simulink model "modulation"  (R2019b)
settings: Solver=ode23t  StartTime=0.0  StopTime=0.008  MaxStep=1e-6  RelTol=1e-3
libraries: powerlib x1
settings Model: Creator=Lenovo  LastModifiedBy=Lenovo

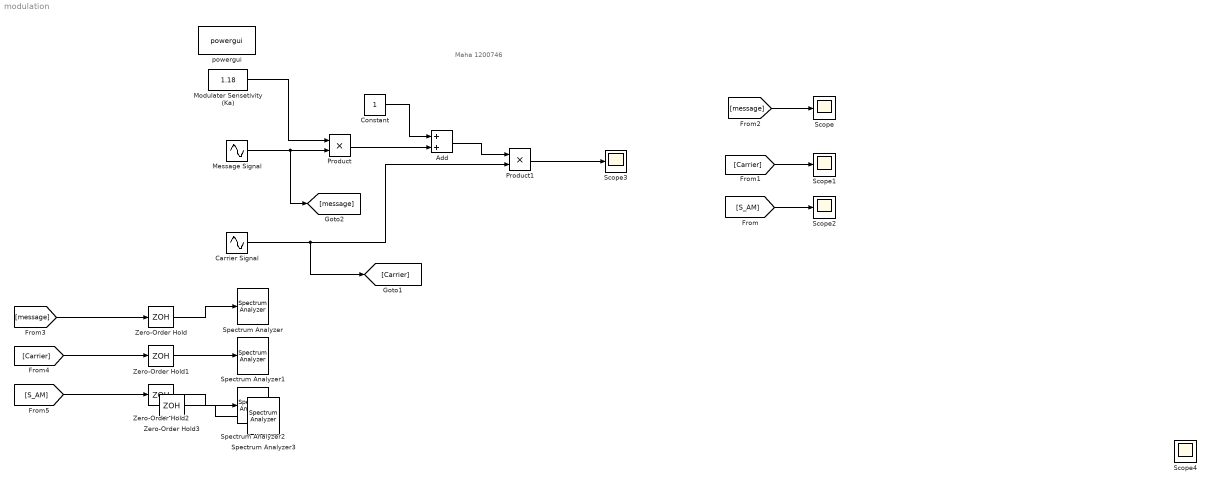
== system modulation ==
  note: Maha 1200746
  Add : Sum
  Carrier Signal : Sin  Frequency=2*pi*15000  SampleTime=0
  Constant : Constant
  Message Signal : Sin  Amplitude=0.85  Frequency=2*pi*1000  SampleTime=0
  Modulater Sensetivity (Ka) : Constant  Value=1.18
  Product : Product
  Product1 : Product
  Scope{,1..4} (5 alike) : Scope
  Spectrum Analyzer{,1..3} (4 alike) : SpectrumAnalyzer
  Zero-Order Hold : ZeroOrderHold  SampleTime=1/(10*1e3)
  Zero-Order Hold1 : ZeroOrderHold  SampleTime=1/(10*15e3)
  Zero-Order Hold2 : ZeroOrderHold  SampleTime=1/(10*15e3)
  Zero-Order Hold3 : ZeroOrderHold  SampleTime=1/(10*15e3)
  powergui : powerlib/powergui  Priority=1  SimulationMode=Continuous  SampleTime=50e-6  frequency=60  Iterations=50  frequencyindice=60  Pbase=100e6  ErrMax=1e-4  UnitsV=kV  UnitsW=MW  buscounter=0  FunctionMessages=off  echomessages=off  EnableUseOfTLC=off  CurrentSourceSwitches=off  DisableSnubberDevices=off  DisableRonSwitches=off  DisableVfSwitches=off  DisplayEquations=off  AutomaticDiscreteSolvers=off  SolverType=Tustin/Backward Euler (TBE)  Interpol=off  ExternalGateDelay=off  methode=off  Ts=100  x0status=blocks  SPID=on  SwTol=0  HookPort=off  NonlinearTolerance=1e-4  nMaxIteration=100  ContinueOnMaxIteration=off  RestoreLinks=warning  ResistiveCurrentMeasurement=off  Frange=[0:2:500]  Ylog=off  Xlog=on  ShowGrid=off  save=off  variable=ZData  structure=0  ZoomFFT=off  StartTime=0.0  cycles=1  DisplayStyle=1  fundamental=60  FreqAxis=off  MaxFrequency=1000  frequencyindicesteady=1  RmsSteady=1  display=off
      settings: SourceProductName=Simscape Electrical
  wires:
  Message Signal/1 -> [message], Product/2
  Modulater Sensetivity (Ka)/1 -> Product/1
  Product/1 -> Add/2
  Constant/1 -> Add/1
  Add/1 -> Product1/1
  Carrier Signal/1 -> [Carrier], Product1/2
  [message] -> Zero-Order Hold/1
  [Carrier] -> Zero-Order Hold1/1
  [S_AM] -> Zero-Order Hold2/1
  Zero-Order Hold2/1 -> Spectrum Analyzer2/1
  Zero-Order Hold1/1 -> Spectrum Analyzer1/1
  Zero-Order Hold/1 -> Spectrum Analyzer/1
  [message] -> Scope/1
  [Carrier] -> Scope1/1
  [S_AM] -> Scope2/1
  Zero-Order Hold3/1 -> Spectrum Analyzer3/1
  ? -> Zero-Order Hold3/1
  Product1/1 -> Scope3/1
